simulink model "closed_loop"  (R2017b)
settings: Solver=VariableStepAuto  StartTime=0.0  StopTime=10  FixedStep=1/500  RelTol=1e-3  AbsTol=1e-3
model workspace: external: MATLAB File params.m (data not in the file)
values from neighbouring files (symbols this model uses):
  b = 2.75e-11    [setup_lqr.m]
  g = 9.82    [setup_lqr.m]
  k = 1e-9    (= 1e-09)    [setup_lqr.m]
  m = 0.027    [setup_lqr.m]
undefined symbols (not defined in the file or in its folder): sensor_position
libraries: nesl_utility x9, simulink x3, simulink_extras x2
settings Model: Creator=Jocke  LastModifiedBy=viktor
settings OptimizationCC: UseDivisionForNetSlopeComputation=on
settings RTWCC: Toolchain=GNU gcc/g++ v4.4.x | gmake (64-bit Linux)
settings CodeAppCC: StateflowObjectComments=on
settings SimscapeCC: SimscapeNormalizeSystem=off  SimscapeLogType=all  SimscapeLogDataHistory=10000

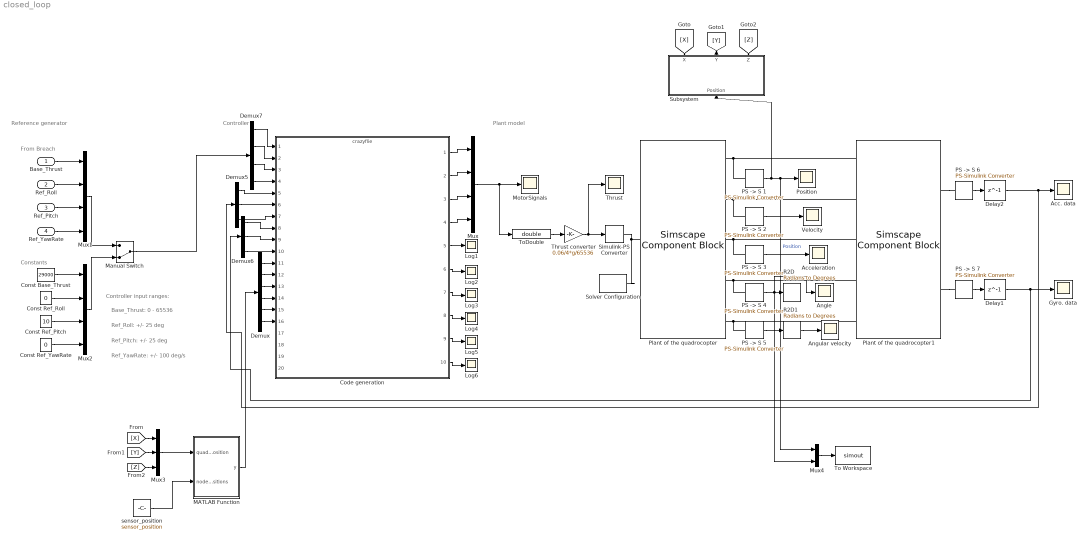
== system closed_loop ==
  note: From Breach
  note: Plant model
  note: Controller
  note: Constants
  note: Reference generator
  note: Ref_Roll: +/- 25 deg
  note: Base_Thrust: 0 - 65536
  note: Ref_Pitch: +/- 25 deg
  note: Ref_YawRate: +/- 100 deg/s
  note: Controller input ranges:
  Base_Thrust : Inport  OutDataTypeStr=double
  Ref_Roll : Inport  Port=2  OutDataTypeStr=double
  Ref_Pitch : Inport  Port=3  OutDataTypeStr=double
  Ref_YawRate : Inport  Port=4  OutDataTypeStr=double
  Acc. data : Scope
  Acceleration : Scope
  Angle : Scope
  Angular velocity : Scope
  Code generation : ModelReference  ModelNameDialog=crazyflie.slx  SimulationMode=Normal  ModelReferenceVersion=1.520
  Const Base_Thrust : Constant  Value=29000
  Const Ref_Pitch : Constant  Value=10
  Const Ref_Roll : Constant  Value=0
  Const Ref_YawRate : Constant  Value=0
  Delay1 : Delay  DelayLength=1
  Delay2 : Delay  DelayLength=1
  Demux : Demux  Outputs=6
  Demux5 : Demux  Outputs=3
  Demux6 : Demux  Outputs=3
  Demux7 : Demux
  Gyro. data : Scope
  Log{1..6} (6 alike) : Scope
  MATLAB Function : MATLAB Function  TreatAsAtomicUnit=on
  Manual Switch : ManualSwitch  CurrentSetting=0
  MotorSignals : Scope
  Mux : Mux
  Mux1 : Mux
  Mux2 : Mux
  Mux3 : Mux  Inputs=3
  Mux4 : Mux  Inputs=2
  PS -> S {1..7} (7 alike) : nesl_utility/PS-Simulink Converter  PhysicalDomain=network_engine_domain  SubClassName=ps_output  LeftPortType=input  RightPortType=output  PseudoPeriodic=off  Frequencies=[]  Unit=1  AffineConversion=off
  Plant of the quadrocopter : SimscapeComponentBlock  SourceFile=plant  ComponentPath=plant  ComponentVariants=plant  ComponentVariantNames=plant  ClassName=plant  SchemaVersion=1  m=m kg  g=g m/s^2  d=d m  k=k kg*m^2  b=b m*kg
      settings: CopyFcn=simscape.engine.sli.internal.componentblockcallback(gcbh,'COPY')  PreCopyFcn=simscape.engine.sli.internal.componentblockcallback(gcbh,'PRECOPY')  PreDeleteFcn=simscape.engine.sli.internal.componentblockcallback(gcbh,'PREDELETE')
      mask Type: Plant of quadrocopter
      mask Display:
      | disp('Simscape\n\n\n')
      | disp('\n\n\nplant');
      | color('red');
      | port_label('RConn', 5,'Angular velocity');
      | port_label('RConn', 4,'Angle');
      | port_label('RConn', 3,'Acceleration');
      | port_label('RConn', 2,'Velocity');
      | port_label('RConn', 1,'Position');
      | port_label('LConn', 1,'Thrust');
  Plant of the quadrocopter1 : SimscapeComponentBlock  SourceFile=sensors  ComponentPath=sensors  ComponentVariants=sensors  ComponentVariantNames=sensors  ClassName=sensors  SchemaVersion=1  m=m kg  g=g m/s^2  d=d m  k=k  b=b
      settings: CopyFcn=simscape.engine.sli.internal.componentblockcallback(gcbh,'COPY')  PreCopyFcn=simscape.engine.sli.internal.componentblockcallback(gcbh,'PRECOPY')  PreDeleteFcn=simscape.engine.sli.internal.componentblockcallback(gcbh,'PREDELETE')
      mask Type: Plant of quadrocopter
      mask Display:
      | disp('Simscape\n\n\n')
      | disp('\n\n\nsensors');
      | color('red');
      | port_label('RConn', 2,'Gyroscope');
      | port_label('RConn', 1,'Accelerometer');
      | port_label('LConn', 5,'Angular velocity');
      | port_label('LConn', 4,'Angle');
      | port_label('LConn', 3,'Acceleration');
      | port_label('LConn', 2,'Velocity');
      | port_label('LConn', 1,'Position');
  Position : Scope
  R2D : simulink_extras/Transformations/Radians to Degrees
  R2D1 : simulink_extras/Transformations/Radians to Degrees
  Simulink-PS Converter : nesl_utility/Simulink-PS Converter  PhysicalDomain=network_engine_domain  SubClassName=ps_input  LeftPortType=input  RightPortType=output  PseudoPeriodic=off  Frequencies=[]  NoiseDistribution=none  NoiseParameters=[]  Unit=1  AffineConversion=off  FilteringAndDerivatives=zero  SimscapeFilterOrder=1  InputFilterTimeConstant=0.001  UdotUserProvided=1
  Solver Configuration : nesl_utility/Solver Configuration  PhysicalDomain=network_engine_domain  SubClassName=solver  LeftPortType=input  RightPortType=generic  Accelerate=off  Tones=[]  Harmonics=[]  SimulateNoise=off  Profile=off  UseLocalSampling=off  EnableSwitchedLinearOptims=on  FrequencyDomain=off  UseCCode=off  RelTol=0.001  AbsTol=1e-06  MinStep=1e-09  ToWorkspace=off  RevertToSquareIcSolve=off  NumHomotopyIterations=100  PhasorMode=off  PhasorModeNumHarmonics=1  DoDC=off  ResidualTolerance=1e-09  UseLocalSolver=off  LocalSolverChoice=NE_BACKWARD_EULER_ADVANCER  LocalSolverSampleTime=0.001  DoFixedCost=off  MaxNonlinIter=3  MaxModeIter=2  LinearAlgebra=Sparse  DelaysMemoryBudget=1024  AutomaticFiltering=on  FilteringTimeConstant=0.001
  Subsystem : Subsystem
  Thrust : Scope
  Thrust converter : Gain  Gain=0.06/4*g/65536
  To Workspace : ToWorkspace  VariableName=simout  SaveFormat=Timeseries  SampleTime=-1
  ToDouble : DataTypeConversion  OutDataTypeStr=double  RndMeth=Round  SaturateOnIntegerOverflow=on
  Velocity : Scope
  sensor_position : Constant  Value=sensor_position
  wires:
  Code generation/1 -> Mux/1
  Code generation/4 -> Mux/4
  Code generation/3 -> Mux/3
  Code generation/2 -> Mux/2
  Demux5/1 -> Code generation/5
  Demux5/2 -> Code generation/6
  Demux5/3 -> Code generation/7
  Demux6/1 -> Code generation/8
  Demux6/2 -> Code generation/9
  Demux6/3 -> Code generation/10
  "PS -> S 7"/1 -> Delay1/1
  Code generation/5 -> Log1/1
  Code generation/6 -> Log2/1
  Code generation/7 -> Log3/1
  Code generation/8 -> Log4/1
  Code generation/9 -> Log5/1
  Code generation/10 -> Log6/1
  Mux/1 -> MotorSignals/1, ToDouble/1
  Base_Thrust/1 -> Mux1/1
  Ref_Roll/1 -> Mux1/2
  Ref_Pitch/1 -> Mux1/3
  Ref_YawRate/1 -> Mux1/4
  Mux1/1 -> Manual Switch/1
  Const Base_Thrust/1 -> Mux2/1
  Const Ref_Roll/1 -> Mux2/2
  Const Ref_Pitch/1 -> Mux2/3
  Const Ref_YawRate/1 -> Mux2/4
  Mux2/1 -> Manual Switch/2
  Manual Switch/1 -> Demux7/1
  Demux7/1 -> Code generation/1
  Demux7/2 -> Code generation/2
  Demux7/3 -> Code generation/3
  Demux7/4 -> Code generation/4
  R2D1/1 -> Angular velocity/1
  ToDouble/1 -> Thrust converter/1
  Thrust converter/1 -> Thrust/1, Simulink-PS Converter/1
  "PS -> S 1"/1 -> Mux4/1, Position/1, Subsystem/1(Position)  "Position"
  "PS -> S 5"/1 -> R2D1/1
  "PS -> S 4"/1 -> Mux4/2, Angle/1, R2D/1
  "PS -> S 3"/1 -> Acceleration/1
  "PS -> S 2"/1 -> Velocity/1
  Delay1/1 -> Gyro. data/1, Demux6/1
  "PS -> S 6"/1 -> Delay2/1
  Delay2/1 -> Acc. data/1, Demux5/1
  Subsystem/3(Z) -> [Z]
  Subsystem/2(Y) -> [Y]
  Subsystem/1(X) -> [X]
  Mux3/1 -> MATLAB Function/1(quadPosition)
  [Y] -> Mux3/2
  [X] -> Mux3/1
  [Z] -> Mux3/3
  sensor_position/1 -> MATLAB Function/2(nodePositions)
  Demux/2 -> Code generation/12
  Demux/6 -> Code generation/16
  Demux/1 -> Code generation/11
  Demux/3 -> Code generation/13
  Demux/4 -> Code generation/14
  Demux/5 -> Code generation/15
  MATLAB Function/1(y) -> Demux/1
  Mux4/1 -> To Workspace/1
  connections:
  Simulink-PS Converter/RConn1 -- Solver Configuration/RConn1 -- Plant of the quadrocopter/LConn1
  Plant of the quadrocopter1/LConn1 -- "PS -> S 1"/LConn1 -- Plant of the quadrocopter/RConn1
  Plant of the quadrocopter1/LConn2 -- "PS -> S 2"/LConn1 -- Plant of the quadrocopter/RConn2
  Plant of the quadrocopter1/LConn3 -- "PS -> S 3"/LConn1 -- Plant of the quadrocopter/RConn3
  Plant of the quadrocopter1/LConn4 -- "PS -> S 4"/LConn1 -- Plant of the quadrocopter/RConn4
  Plant of the quadrocopter1/LConn5 -- "PS -> S 5"/LConn1 -- Plant of the quadrocopter/RConn5
  Plant of the quadrocopter1/RConn1 -- "PS -> S 6"/LConn1
  Plant of the quadrocopter1/RConn2 -- "PS -> S 7"/LConn1

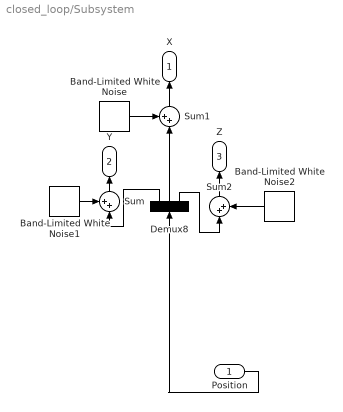
== system closed_loop/Subsystem ==
  Position : Inport
  Band-Limited White Noise : simulink/Sources/Band-Limited White Noise  Cov=[0.1]  Ts=0.1  seed=[2325226241]
  Band-Limited White Noise1 : simulink/Sources/Band-Limited White Noise  Cov=[0.1]  Ts=0.1  seed=[23341]
  Band-Limited White Noise2 : simulink/Sources/Band-Limited White Noise  Cov=[0.1]  Ts=0.1  seed=[23364641]
  Demux8 : Demux  Outputs=3
  Sum : Sum  Inputs=++|
  Sum1 : Sum  Inputs=++|
  Sum2 : Sum  Inputs=|++
  X : Outport
  Y : Outport  Port=2
  Z : Outport  Port=3
  wires:
  Demux8/1 -> Sum/2
  Band-Limited White Noise2/1 -> Sum2/2
  Demux8/3 -> Sum2/1
  Band-Limited White Noise/1 -> Sum1/1
  Band-Limited White Noise1/1 -> Sum/1
  Sum2/1 -> Z/1
  Demux8/2 -> Sum1/2
  Position/1 -> Demux8/1
  Sum1/1 -> X/1
  Sum/1 -> Y/1

== matlab function closed_loop/MATLAB Function ==
  data: quadPosition input; y output; nodePositions input
function y = fcn(quadPosition, nodePositions)

y = simulateLPSoutput(quadPosition, nodePositions);
